simulink model "GlwLmp"  (R2016b)
settings: Solver=VariableStepAuto  StartTime=0.0  StopTime=10.0  RelTol=1e-3
settings Model: Creator=jiakui  LastModifiedBy=jiakui

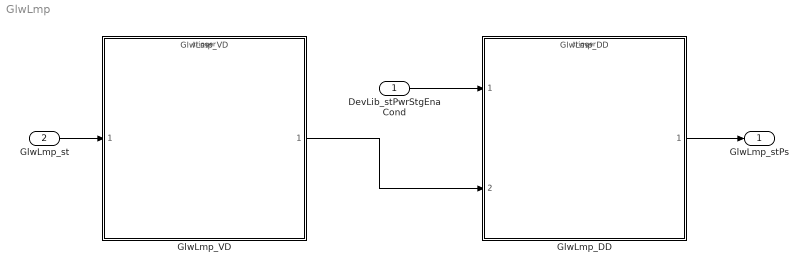
== system GlwLmp ==
  DevLib_stPwrStgEnaCond : Inport  Description=Control unit status relevant to power stage deactivation/error diagnosis  OutMin=0  OutMax=65535  OutDataTypeStr=State_uint16
  GlwLmp_st : Inport  Description=Glow lamp status  Port=2  OutMin=0  OutMax=1  OutDataTypeStr=boolean
  GlwLmp_DD : ModelReference  ModelNameDialog=GlwLmp_DD  SimulationMode=Normal  ModelReferenceVersion=1.5  TriggerPortName=function  TriggerPortTriggerType=function-call  TriggerPortStatesWhenEnabling=held
  GlwLmp_VD : ModelReference  ModelNameDialog=GlwLmp_VD  SimulationMode=Normal  ModelReferenceVersion=1.3  TriggerPortName=function  TriggerPortTriggerType=function-call  TriggerPortStatesWhenEnabling=held
  GlwLmp_stPs : Outport  Description=Digital output to the actuator after diagnosis  OutMin=0  OutMax=1  OutDataTypeStr=boolean
  wires:
  DevLib_stPwrStgEnaCond/1 -> GlwLmp_DD/1
  GlwLmp_VD/1 -> GlwLmp_DD/2
  GlwLmp_DD/1 -> GlwLmp_stPs/1
  GlwLmp_st/1 -> GlwLmp_VD/1
